simulink model "Identificare"  (R2023b)
settings: Solver=FixedStepAuto  StartTime=0.0  StopTime=1000  FixedStep=0.01  RelTol=1e-3
values from neighbouring files (symbols this model uses):
  A = 332.5    [CodDatepersonale.m]    (also in CodProiect.m; untitled.m; untitled2.m = [O I; O O]; untitled22.m)
  C = 7.4    [CodDatepersonale.m]    (also in CodProiect.m = 9; untitled.m; untitled22.m = 9)
  k = 0.036    [CodDatepersonale.m]    (also in CodProiect.m = 0.035; untitled.m; untitled22.m = 0.035)
  k11 = k2^2+4*(k-k3)*k1    (= 0.0915786)    [CodDatepersonale.m]    (also in CodProiect.m = 0.0933546; untitled.m = 0.0959706; untitled22.m = 0.0890826)
  k12 = 4*(k-k3)*Pv    (= 0.2928)    [CodDatepersonale.m]    (also in CodProiect.m = 0.2848; untitled.m; untitled22.m = 0.2848)
  k13 = 2*(k-k3)    (= 0.0732)    [CodDatepersonale.m]    (also in CodProiect.m = 0.0712; untitled.m; untitled22.m = 0.0712)
  k2 = -0.015    [CodDatepersonale.m]    (also in CodProiect.m; untitled.m; untitled22.m)
  keta = 8*10^(-5)    (= 8e-05)    [CodDatepersonale.m]    (also in CodProiect.m; untitled.m; untitled22.m)
settings Model: Creator=Daniela  LastModifiedBy=Daniela
settings SolverCC: MaxConsecutiveMinStep=10

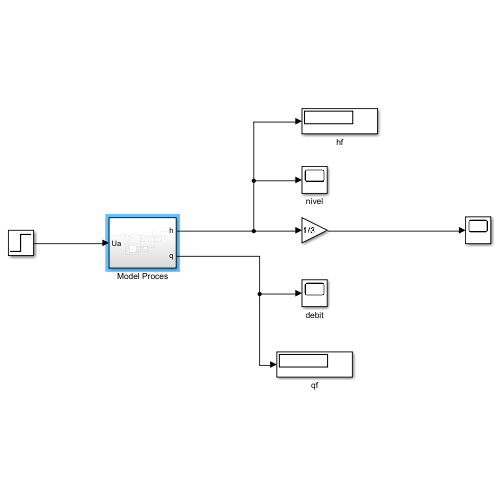
[thumbnail: Simulink's stored preview of the top-level diagram]
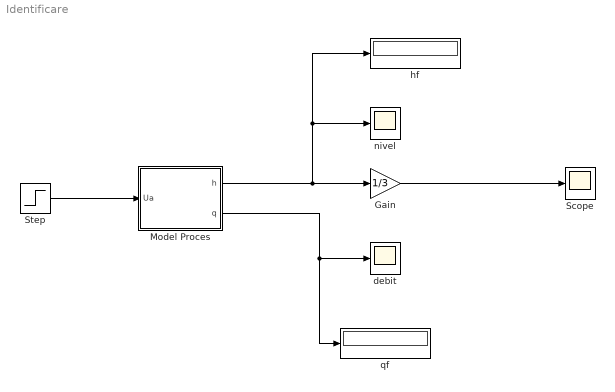
== system Identificare ==
  Gain : Gain  Gain=1/3
  Model Proces : Subsystem
  Scope : Scope
  Step : Step  Time=0  After=6.1  SampleTime=0
  debit : Scope
  hf : Display
  nivel : Scope
  qf : Display
  wires:
  Model Proces/1(h) -> hf/1, nivel/1, Gain/1
  Gain/1 -> Scope/1
  Step/1 -> Model Proces/1(Ua)
  Model Proces/2(q) -> qf/1, debit/1

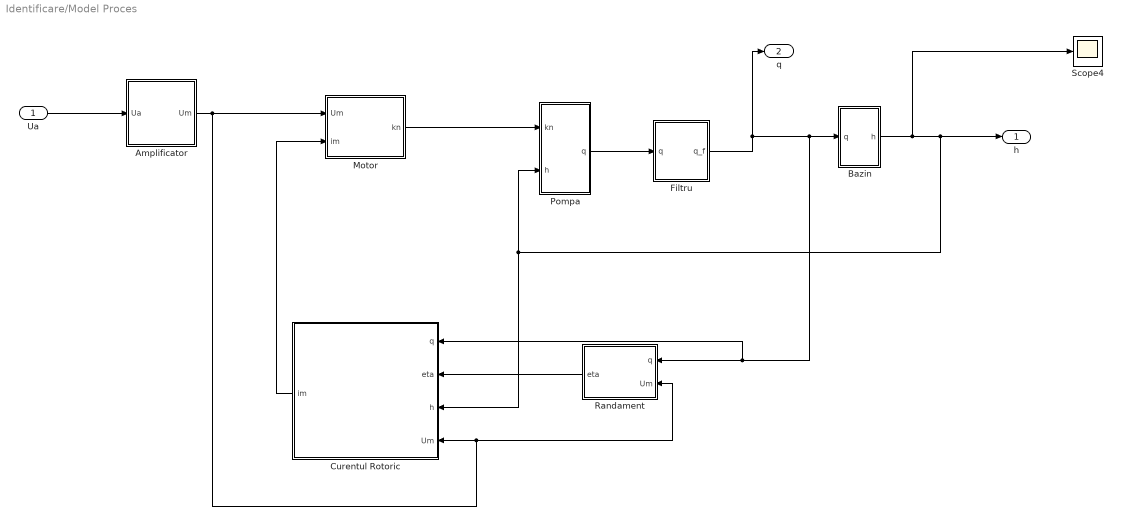
== system Identificare/Model Proces ==
  Ua : Inport
  Amplificator : Subsystem
  Bazin : Subsystem
  Curentul Rotoric : Subsystem
  Filtru : Subsystem
  Motor : Subsystem
  Pompa : Subsystem
  Randament : Subsystem
  Scope4 : Scope
  h : Outport
  q : Outport  Port=2
  wires:
  Amplificator/1(Um) -> Motor/1(Um), Randament/2(Um), Curentul Rotoric/4(Um)
  Filtru/1(q_f) -> Bazin/1(q), Randament/1(q), Curentul Rotoric/1(q), q/1
  Curentul Rotoric/1(im) -> Motor/2(im)
  Bazin/1(h) -> Scope4/1, h/1, Curentul Rotoric/3(h), Pompa/2(h)
  Motor/1(kn) -> Pompa/1(kn)
  Pompa/1(q) -> Filtru/1(q)
  Ua/1 -> Amplificator/1(Ua)
  Randament/1(eta) -> Curentul Rotoric/2(eta)

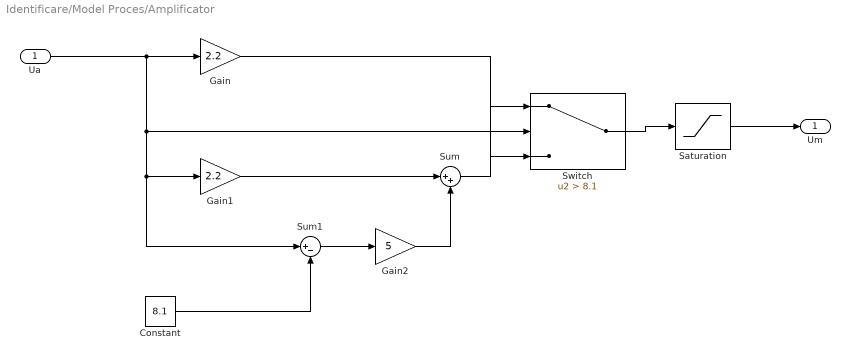
== system Identificare/Model Proces/Amplificator ==
  Ua : Inport
  Constant : Constant  Value=8.1
  Gain : Gain  Gain=2.2
  Gain1 : Gain  Gain=2.2
  Gain2 : Gain  Gain=5
  Saturation : Saturate  UpperLimit=22  LowerLimit=0  ZeroCross=off
  Sum : Sum  Inputs=|++
  Sum1 : Sum  Inputs=|+-
  Switch : Switch  Criteria=u2 > Threshold  Threshold=8.1  SaturateOnIntegerOverflow=off  InputSameDT=off
  Um : Outport
  wires:
  Switch/1 -> Saturation/1
  Ua/1 -> Sum1/1, Gain1/1, Switch/2, Gain/1
  Constant/1 -> Sum1/2
  Sum1/1 -> Gain2/1
  Gain/1 -> Switch/3
  Sum/1 -> Switch/1
  Gain1/1 -> Sum/1
  Gain2/1 -> Sum/2
  Saturation/1 -> Um/1

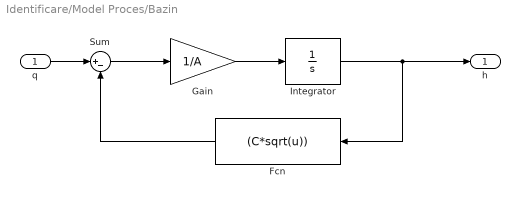
== system Identificare/Model Proces/Bazin ==
  q : Inport
  Fcn : Fcn  Expr=(C*sqrt(u))
  Gain : Gain  Gain=1/A
  Integrator : Integrator  InitialCondition=16.53
  Sum : Sum  Inputs=|+-
  h : Outport
  wires:
  Integrator/1 -> h/1, Fcn/1
  Sum/1 -> Gain/1
  Gain/1 -> Integrator/1
  Fcn/1 -> Sum/2
  q/1 -> Sum/1

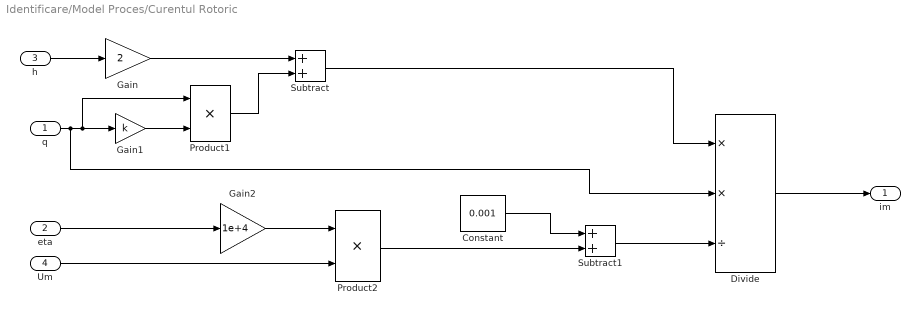
== system Identificare/Model Proces/Curentul Rotoric ==
  q : Inport
  eta : Inport  Port=2
  h : Inport  Port=3
  Um : Inport  Port=4
  Constant : Constant  Value=0.001
  Divide : Product  Inputs=**/
  Gain : Gain  Gain=2
  Gain1 : Gain  Gain=k
  Gain2 : Gain  Gain=1e+4
  Product1 : Product
  Product2 : Product
  Subtract : Sum
  Subtract1 : Sum
  im : Outport
  wires:
  Product1/1 -> Subtract/2
  Um/1 -> Product2/2
  q/1 -> Gain1/1, Product1/1, Divide/2
  Subtract/1 -> Divide/1
  Divide/1 -> im/1
  Subtract1/1 -> Divide/3
  Gain2/1 -> Product2/1
  h/1 -> Gain/1
  Gain/1 -> Subtract/1
  Gain1/1 -> Product1/2
  eta/1 -> Gain2/1
  Product2/1 -> Subtract1/2
  Constant/1 -> Subtract1/1

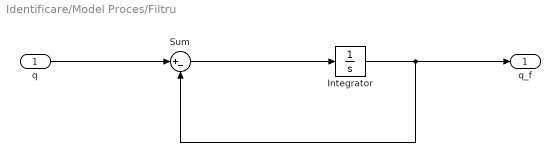
== system Identificare/Model Proces/Filtru ==
  q : Inport
  Integrator : Integrator  InitialCondition=30.22
  Sum : Sum  Inputs=|+-
  q_f : Outport
  wires:
  Integrator/1 -> q_f/1, Sum/2
  q/1 -> Sum/1
  Sum/1 -> Integrator/1

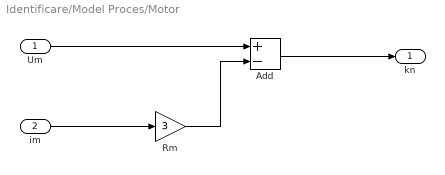
== system Identificare/Model Proces/Motor ==
  Um : Inport
  im : Inport  Port=2
  Add : Sum  Inputs=+-
  Rm : Gain  Gain=3
  kn : Outport
  wires:
  im/1 -> Rm/1
  Add/1 -> kn/1
  Um/1 -> Add/1
  Rm/1 -> Add/2

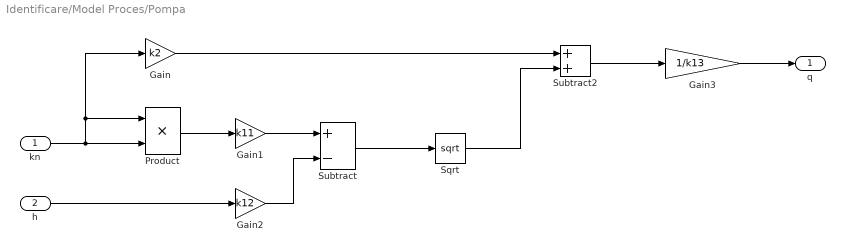
== system Identificare/Model Proces/Pompa ==
  kn : Inport
  h : Inport  Port=2
  Gain : Gain  Gain=k2
  Gain1 : Gain  Gain=k11
  Gain2 : Gain  Gain=k12
  Gain3 : Gain  Gain=1/k13
  Product : Product
  Sqrt : Sqrt
  Subtract : Sum  Inputs=+-
  Subtract2 : Sum
  q : Outport
  wires:
  Subtract/1 -> Sqrt/1
  kn/1 -> Product/2, Product/1, Gain/1
  h/1 -> Gain2/1
  Gain2/1 -> Subtract/2
  Gain/1 -> Subtract2/1
  Product/1 -> Gain1/1
  Gain3/1 -> q/1
  Gain1/1 -> Subtract/1
  Subtract2/1 -> Gain3/1
  Sqrt/1 -> Subtract2/2

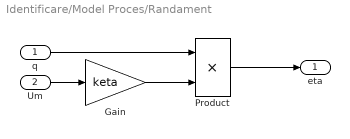
== system Identificare/Model Proces/Randament ==
  q : Inport
  Um : Inport  Port=2
  Gain : Gain  Gain=keta
  Product : Product
  eta : Outport
  wires:
  Gain/1 -> Product/2
  Product/1 -> eta/1
  Um/1 -> Gain/1
  q/1 -> Product/1
